simulink model "uavopen_djian"  (R2022b)
settings: Solver=VariableStepAuto  StartTime=0.0  StopTime=50  RelTol=1e-3
libraries: simulink x1
settings Model: Creator=Zzera  LastModifiedBy=Zzera

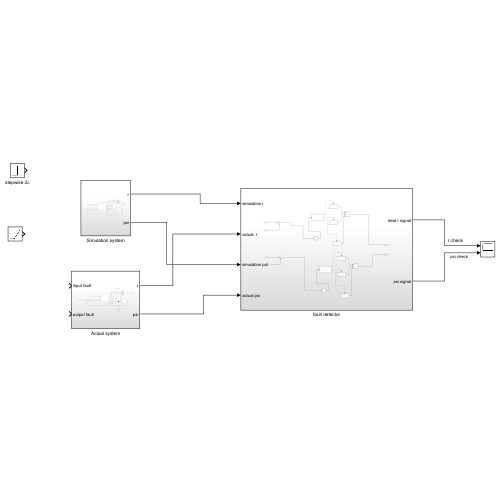
[thumbnail: Simulink's stored preview of the top-level diagram]
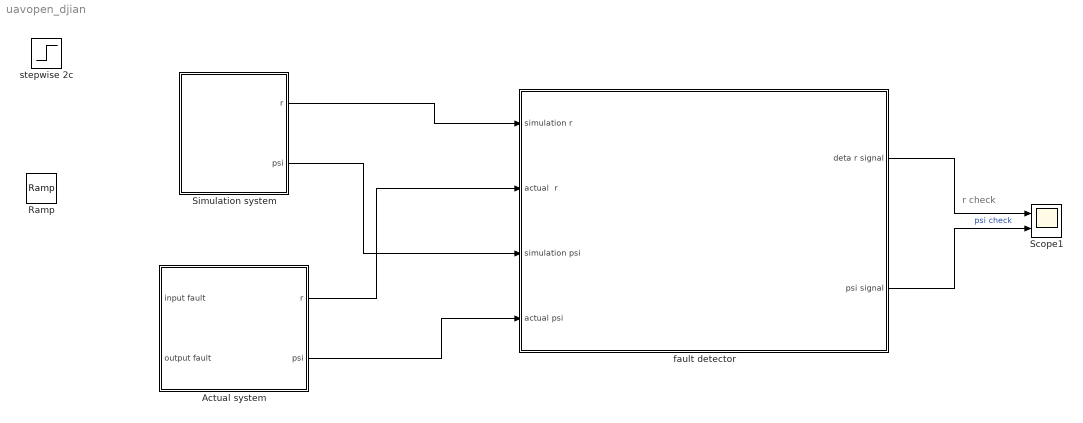
== system uavopen_djian ==
  note: r check
  Actual system : Subsystem
  Ramp : simulink/Sources/Ramp  slope=0.1  start=10  InitialOutput=0
  Scope1 : Scope  NumInputPorts=2
  Simulation system : Subsystem
  fault detector : Subsystem
  stepwise 2c : Step  After=0.2  SampleTime=10
  wires:
  Simulation system/1(" r") -> fault detector/1(simulation r)
  Actual system/1(" r") -> fault detector/2(actual  r)
  Simulation system/2(psi) -> fault detector/3(simulation psi)
  Actual system/2(psi) -> fault detector/4(actual psi)
  fault detector/1(deta r signal) -> Scope1/1
  fault detector/2(psi signal) -> Scope1/2  "psi check"

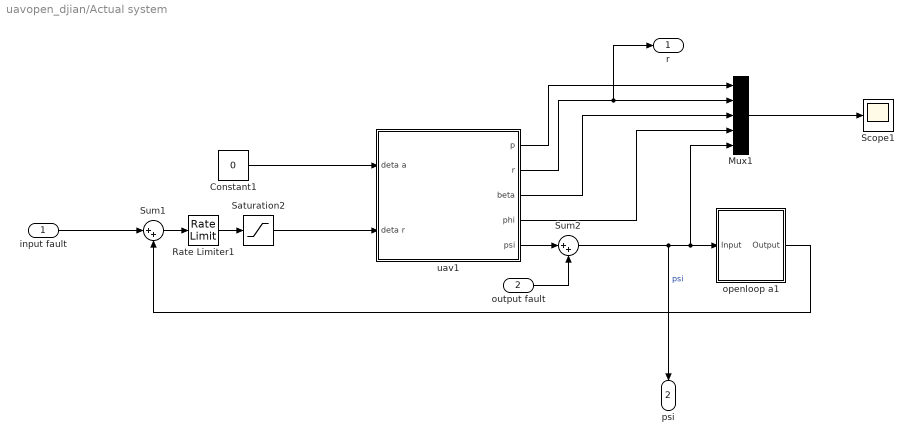
== system uavopen_djian/Actual system ==
  input fault : Inport
  output fault : Inport  Port=2
  Constant1 : Constant  Value=0
  Mux1 : Mux  Inputs=5
  Rate Limiter1 : RateLimiter  RisingSlewLimit=0.3491  FallingSlewLimit=-0.3491
  Saturation2 : Saturate  UpperLimit=1.308  LowerLimit=-1.308
  Scope1 : Scope
  Sum1 : Sum  Inputs=|++
  Sum2 : Sum  Inputs=|++
  openloop a1 : Subsystem
  uav1 : Subsystem
  " r" : Outport
  psi : Outport  Port=2
  wires:
  Sum2/1 -> psi/1, Mux1/5, openloop a1/1(Input)  "psi"
  Saturation2/1 -> uav1/2(deta r)
  openloop a1/1(Output) -> Sum1/2
  uav1/2(r) -> " r"/1, Mux1/2
  uav1/4(phi) -> Mux1/4
  Rate Limiter1/1 -> Saturation2/1
  uav1/1(p) -> Mux1/1
  output fault/1 -> Sum2/2
  Mux1/1 -> Scope1/1
  Constant1/1 -> uav1/1(deta a)
  uav1/3(beta) -> Mux1/3
  Sum1/1 -> Rate Limiter1/1
  uav1/5(psi) -> Sum2/1
  input fault/1 -> Sum1/1

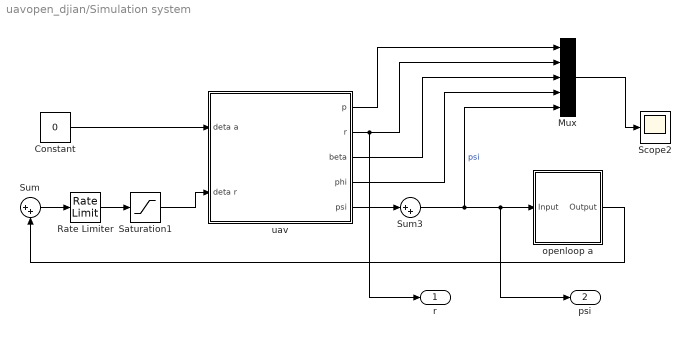
== system uavopen_djian/Simulation system ==
  Constant : Constant  Value=0
  Mux : Mux  Inputs=5
  Rate Limiter : RateLimiter  RisingSlewLimit=0.3491  FallingSlewLimit=-0.3491
  Saturation1 : Saturate  UpperLimit=1.308  LowerLimit=-1.308
  Scope2 : Scope
  Sum : Sum  Inputs=|++
  Sum3 : Sum  Inputs=|++
  openloop a : Subsystem
  uav : Subsystem
  " r" : Outport
  psi : Outport  Port=2
  wires:
  uav/4(phi) -> Mux/4
  uav/5(psi) -> Sum3/1
  Sum3/1 -> psi/1, openloop a/1(Input), Mux/5  "psi"
  Saturation1/1 -> uav/2(deta r)
  uav/2(r) -> " r"/1, Mux/2
  uav/1(p) -> Mux/1
  Rate Limiter/1 -> Saturation1/1
  uav/3(beta) -> Mux/3
  openloop a/1(Output) -> Sum/2
  Mux/1 -> Scope2/1
  Constant/1 -> uav/1(deta a)
  Sum/1 -> Rate Limiter/1

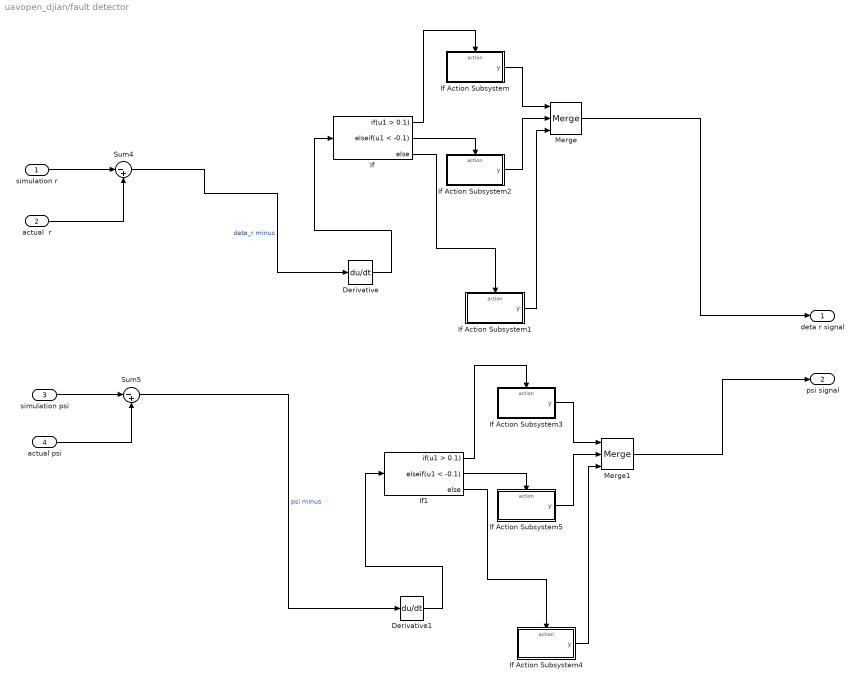
== system uavopen_djian/fault detector ==
  simulation r : Inport
  actual  r : Inport  Port=2
  simulation psi : Inport  Port=3
  actual psi : Inport  Port=4
  Derivative : Derivative
  Derivative1 : Derivative
  If : If  IfExpression=u1 > 0.1  ElseIfExpressions=u1 < -0.1  ZeroCross=off
  If Action Subsystem : Subsystem  TreatAsAtomicUnit=on
  If Action Subsystem1 : Subsystem  TreatAsAtomicUnit=on
  If Action Subsystem2 : Subsystem  TreatAsAtomicUnit=on
  If Action Subsystem3 : Subsystem  TreatAsAtomicUnit=on
  If Action Subsystem4 : Subsystem  TreatAsAtomicUnit=on
  If Action Subsystem5 : Subsystem  TreatAsAtomicUnit=on
  If1 : If  IfExpression=u1 > 0.1  ElseIfExpressions=u1 < -0.1  ZeroCross=off
  Merge : Merge  Inputs=3
  Merge1 : Merge  Inputs=3
  Sum4 : Sum  Inputs=|-+
  Sum5 : Sum  Inputs=|-+
  deta r signal : Outport
  psi signal : Outport  Port=2
  wires:
  If Action Subsystem3/1(y) -> Merge1/1
  If/3 -> If Action Subsystem1/Action
  Derivative/1 -> If/1
  If Action Subsystem/1(y) -> Merge/1
  Derivative1/1 -> If1/1
  If Action Subsystem5/1(y) -> Merge1/2
  If Action Subsystem4/1(y) -> Merge1/3
  simulation r/1 -> Sum4/1
  If1/1 -> If Action Subsystem3/Action
  If1/3 -> If Action Subsystem4/Action
  If1/2 -> If Action Subsystem5/Action
  If/2 -> If Action Subsystem2/Action
  Sum4/1 -> Derivative/1  "deta_r minus"
  Merge1/1 -> psi signal/1
  If/1 -> If Action Subsystem/Action
  If Action Subsystem2/1(y) -> Merge/2
  If Action Subsystem1/1(y) -> Merge/3
  Sum5/1 -> Derivative1/1  "psi minus"
  Merge/1 -> deta r signal/1
  actual  r/1 -> Sum4/2
  simulation psi/1 -> Sum5/1
  actual psi/1 -> Sum5/2

== system uavopen_djian/Actual system/openloop a1 ==
  Input : Inport
  If : If  IfExpression=u1>0.1746  ElseIfExpressions=u1<-0.1745  ShowElse=off
  If Action Subsystem : Subsystem  TreatAsAtomicUnit=on
  If Action Subsystem1 : Subsystem  TreatAsAtomicUnit=on
  Merge : Merge  InitialOutput=[0.3491]
  Output : Outport
  wires:
  Input/1 -> If/1
  If Action Subsystem/1(y) -> Merge/1
  If Action Subsystem1/1(Out1) -> Merge/2
  If/1 -> If Action Subsystem/Action
  If/2 -> If Action Subsystem1/Action
  Merge/1 -> Output/1

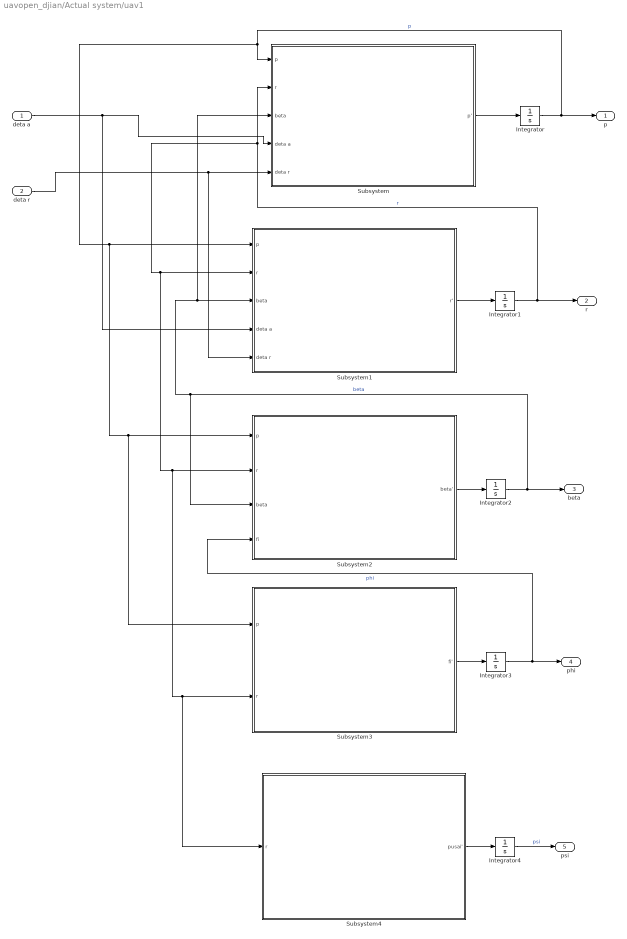
== system uavopen_djian/Actual system/uav1 ==
  deta a : Inport
  deta r : Inport  Port=2
  Integrator{,1..4} (5 alike) : Integrator
  Subsystem : Subsystem
  Subsystem1 : Subsystem
  Subsystem2 : Subsystem
  Subsystem3 : Subsystem
  Subsystem4 : Subsystem
  p : Outport
  r : Outport  Port=2
  beta : Outport  Port=3
  phi : Outport  Port=4
  psi : Outport  Port=5
  wires:
  Integrator4/1 -> psi/1  "psi"
  Integrator3/1 -> phi/1, Subsystem2/4(fi)  "phi"
  Subsystem/1(p') -> Integrator/1
  Subsystem3/1(fi') -> Integrator3/1
  Integrator/1 -> p/1, Subsystem3/1(p), Subsystem2/1(p), Subsystem1/1(p), Subsystem/1(p)  "p"
  Subsystem2/1(beta') -> Integrator2/1
  Integrator1/1 -> r/1, Subsystem/2(r), Subsystem4/1(r), Subsystem3/2(r), Subsystem2/2(r), Subsystem1/2(r)  "r"
  Subsystem4/1(pusai') -> Integrator4/1
  Integrator2/1 -> beta/1, Subsystem2/3(beta), Subsystem/3(beta), Subsystem1/3(beta)  "beta"
  Subsystem1/1(r') -> Integrator1/1
  deta a/1 -> Subsystem1/4(deta a), Subsystem/4(deta a)
  deta r/1 -> Subsystem1/5(deta r), Subsystem/5(deta r)

== system uavopen_djian/Simulation system/openloop a ==
  Input : Inport
  If : If  IfExpression=u1>0.1746  ElseIfExpressions=u1<-0.1745  ShowElse=off
  If Action Subsystem : Subsystem  TreatAsAtomicUnit=on
  If Action Subsystem1 : Subsystem  TreatAsAtomicUnit=on
  Merge : Merge  InitialOutput=[0.3491]
  Output : Outport
  wires:
  Input/1 -> If/1
  If Action Subsystem/1(y) -> Merge/1
  If Action Subsystem1/1(Out1) -> Merge/2
  If/1 -> If Action Subsystem/Action
  If/2 -> If Action Subsystem1/Action
  Merge/1 -> Output/1

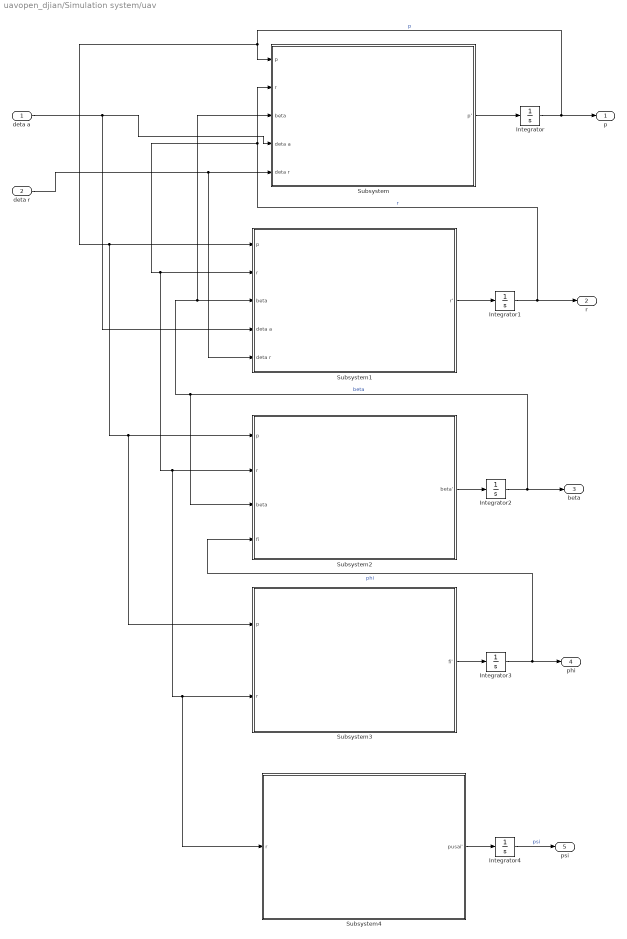
== system uavopen_djian/Simulation system/uav ==
  deta a : Inport
  deta r : Inport  Port=2
  Integrator{,1..4} (5 alike) : Integrator
  Subsystem : Subsystem
  Subsystem1 : Subsystem
  Subsystem2 : Subsystem
  Subsystem3 : Subsystem
  Subsystem4 : Subsystem
  p : Outport
  r : Outport  Port=2
  beta : Outport  Port=3
  phi : Outport  Port=4
  psi : Outport  Port=5
  wires:
  Integrator4/1 -> psi/1  "psi"
  Integrator3/1 -> phi/1, Subsystem2/4(fi)  "phi"
  Subsystem/1(p') -> Integrator/1
  Subsystem3/1(fi') -> Integrator3/1
  Integrator/1 -> p/1, Subsystem3/1(p), Subsystem2/1(p), Subsystem1/1(p), Subsystem/1(p)  "p"
  Subsystem2/1(beta') -> Integrator2/1
  Integrator1/1 -> r/1, Subsystem/2(r), Subsystem4/1(r), Subsystem3/2(r), Subsystem2/2(r), Subsystem1/2(r)  "r"
  Subsystem4/1(pusai') -> Integrator4/1
  Integrator2/1 -> beta/1, Subsystem2/3(beta), Subsystem/3(beta), Subsystem1/3(beta)  "beta"
  Subsystem1/1(r') -> Integrator1/1
  deta a/1 -> Subsystem1/4(deta a), Subsystem/4(deta a)
  deta r/1 -> Subsystem1/5(deta r), Subsystem/5(deta r)

== system uavopen_djian/fault detector/If Action Subsystem ==
  Action Port : ActionPort  ActionPortLabel=if(u1 > 0.1)
  Constant : Constant
  y : Outport
  wires:
  Constant/1 -> y/1

== system uavopen_djian/fault detector/If Action Subsystem1 ==
  Action Port : ActionPort  ActionPortLabel=else
  Constant : Constant  Value=0
  y : Outport
  wires:
  Constant/1 -> y/1

== system uavopen_djian/fault detector/If Action Subsystem2 ==
  Action Port : ActionPort  ActionPortLabel=elseif(u1 < -0.1)
  Constant : Constant
  y : Outport
  wires:
  Constant/1 -> y/1

== system uavopen_djian/fault detector/If Action Subsystem3 ==
  Action Port : ActionPort  ActionPortLabel=if(u1 > 0.1)
  Constant : Constant
  y : Outport
  wires:
  Constant/1 -> y/1

== system uavopen_djian/fault detector/If Action Subsystem4 ==
  Action Port : ActionPort  ActionPortLabel=else
  Constant : Constant  Value=0
  y : Outport
  wires:
  Constant/1 -> y/1

== system uavopen_djian/fault detector/If Action Subsystem5 ==
  Action Port : ActionPort  ActionPortLabel=elseif(u1 < -0.1)
  Constant : Constant
  y : Outport
  wires:
  Constant/1 -> y/1

== system uavopen_djian/Actual system/openloop a1/If Action Subsystem ==
  Action Port : ActionPort  ActionPortLabel=if(u1>0.1746)
  Constant : Constant  Value=-0.3491
  y : Outport
  wires:
  Constant/1 -> y/1

== system uavopen_djian/Actual system/openloop a1/If Action Subsystem1 ==
  Action Port : ActionPort  ActionPortLabel=elseif(u1<-0.1745)
  Constant : Constant  Value=0.3491
  Out1 : Outport
  wires:
  Constant/1 -> Out1/1

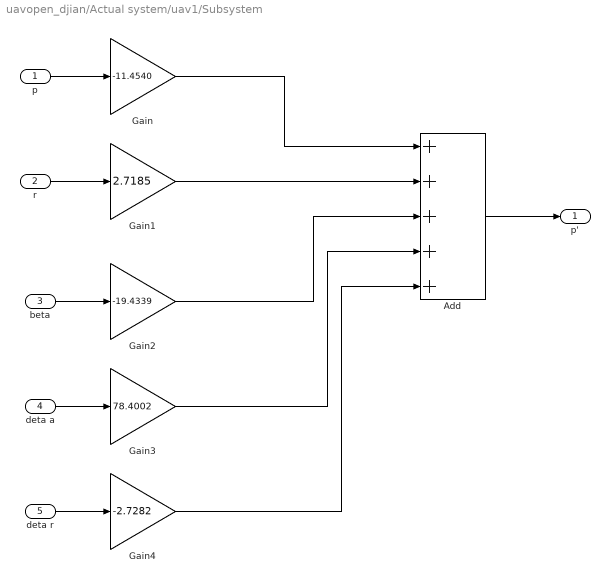
== system uavopen_djian/Actual system/uav1/Subsystem ==
  p : Inport
  r : Inport  Port=2
  beta : Inport  Port=3
  deta a : Inport  Port=4
  deta r : Inport  Port=5
  Add : Sum  Inputs=+++++
  Gain : Gain  Gain=-11.4540
  Gain1 : Gain  Gain=2.7185
  Gain2 : Gain  Gain=-19.4339
  Gain3 : Gain  Gain=78.4002
  Gain4 : Gain  Gain=-2.7282
  p' : Outport
  wires:
  Gain2/1 -> Add/3
  Gain3/1 -> Add/4
  Gain/1 -> Add/1
  Gain1/1 -> Add/2
  Gain4/1 -> Add/5
  p/1 -> Gain/1
  r/1 -> Gain1/1
  beta/1 -> Gain2/1
  deta a/1 -> Gain3/1
  deta r/1 -> Gain4/1
  Add/1 -> p'/1

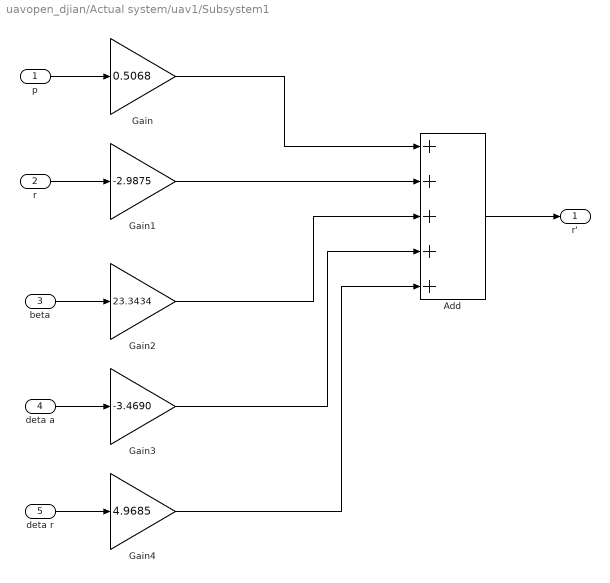
== system uavopen_djian/Actual system/uav1/Subsystem1 ==
  p : Inport
  r : Inport  Port=2
  beta : Inport  Port=3
  deta a : Inport  Port=4
  deta r : Inport  Port=5
  Add : Sum  Inputs=+++++
  Gain : Gain  Gain=0.5068
  Gain1 : Gain  Gain=-2.9875
  Gain2 : Gain  Gain=23.3434
  Gain3 : Gain  Gain=-3.4690
  Gain4 : Gain  Gain=4.9685
  r' : Outport
  wires:
  p/1 -> Gain/1
  Gain4/1 -> Add/5
  Gain1/1 -> Add/2
  Gain/1 -> Add/1
  Gain2/1 -> Add/3
  beta/1 -> Gain2/1
  Gain3/1 -> Add/4
  deta a/1 -> Gain3/1
  Add/1 -> r'/1
  deta r/1 -> Gain4/1
  r/1 -> Gain1/1

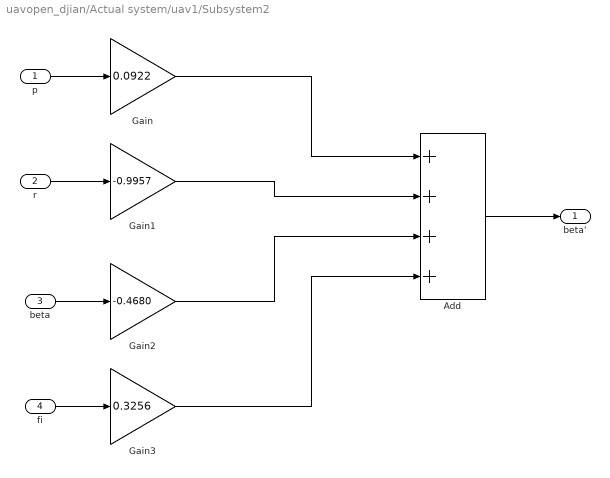
== system uavopen_djian/Actual system/uav1/Subsystem2 ==
  p : Inport
  r : Inport  Port=2
  beta : Inport  Port=3
  fi : Inport  Port=4
  Add : Sum  Inputs=++++
  Gain : Gain  Gain=0.0922
  Gain1 : Gain  Gain=-0.9957
  Gain2 : Gain  Gain=-0.4680
  Gain3 : Gain  Gain=0.3256
  beta' : Outport
  wires:
  p/1 -> Gain/1
  Gain1/1 -> Add/2
  Gain/1 -> Add/1
  Gain2/1 -> Add/3
  beta/1 -> Gain2/1
  Gain3/1 -> Add/4
  fi/1 -> Gain3/1
  Add/1 -> beta'/1
  r/1 -> Gain1/1

== system uavopen_djian/Actual system/uav1/Subsystem3 ==
  p : Inport
  r : Inport  Port=2
  Add : Sum
  Gain : Gain
  Gain1 : Gain  Gain=0.0926
  fi' : Outport
  wires:
  p/1 -> Gain/1
  Gain1/1 -> Add/2
  Gain/1 -> Add/1
  Add/1 -> fi'/1
  r/1 -> Gain1/1

== system uavopen_djian/Actual system/uav1/Subsystem4 ==
  r : Inport
  Gain1 : Gain
  pusai' : Outport
  wires:
  r/1 -> Gain1/1
  Gain1/1 -> pusai'/1

== system uavopen_djian/Simulation system/openloop a/If Action Subsystem ==
  Action Port : ActionPort  ActionPortLabel=if(u1>0.1746)
  Constant : Constant  Value=-0.3491
  y : Outport
  wires:
  Constant/1 -> y/1

== system uavopen_djian/Simulation system/openloop a/If Action Subsystem1 ==
  Action Port : ActionPort  ActionPortLabel=elseif(u1<-0.1745)
  Constant : Constant  Value=0.3491
  Out1 : Outport
  wires:
  Constant/1 -> Out1/1

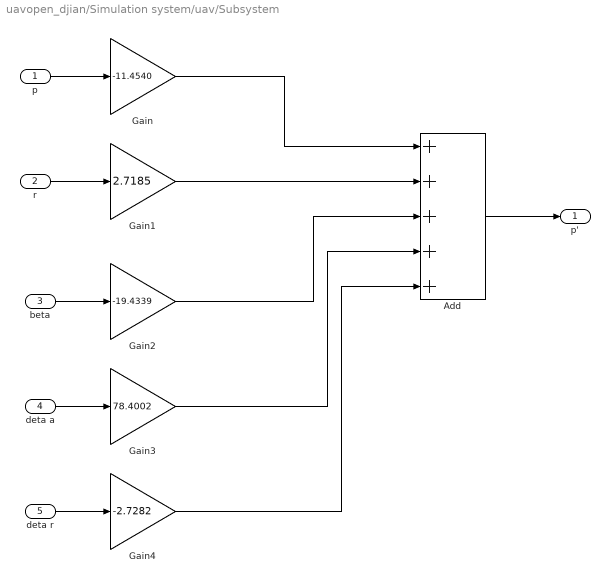
== system uavopen_djian/Simulation system/uav/Subsystem ==
  p : Inport
  r : Inport  Port=2
  beta : Inport  Port=3
  deta a : Inport  Port=4
  deta r : Inport  Port=5
  Add : Sum  Inputs=+++++
  Gain : Gain  Gain=-11.4540
  Gain1 : Gain  Gain=2.7185
  Gain2 : Gain  Gain=-19.4339
  Gain3 : Gain  Gain=78.4002
  Gain4 : Gain  Gain=-2.7282
  p' : Outport
  wires:
  Gain2/1 -> Add/3
  Gain3/1 -> Add/4
  Gain/1 -> Add/1
  Gain1/1 -> Add/2
  Gain4/1 -> Add/5
  p/1 -> Gain/1
  r/1 -> Gain1/1
  beta/1 -> Gain2/1
  deta a/1 -> Gain3/1
  deta r/1 -> Gain4/1
  Add/1 -> p'/1

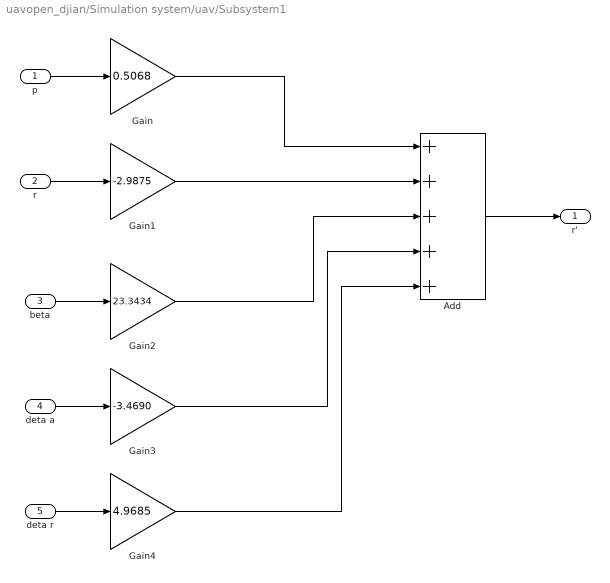
== system uavopen_djian/Simulation system/uav/Subsystem1 ==
  p : Inport
  r : Inport  Port=2
  beta : Inport  Port=3
  deta a : Inport  Port=4
  deta r : Inport  Port=5
  Add : Sum  Inputs=+++++
  Gain : Gain  Gain=0.5068
  Gain1 : Gain  Gain=-2.9875
  Gain2 : Gain  Gain=23.3434
  Gain3 : Gain  Gain=-3.4690
  Gain4 : Gain  Gain=4.9685
  r' : Outport
  wires:
  p/1 -> Gain/1
  Gain4/1 -> Add/5
  Gain1/1 -> Add/2
  Gain/1 -> Add/1
  Gain2/1 -> Add/3
  beta/1 -> Gain2/1
  Gain3/1 -> Add/4
  deta a/1 -> Gain3/1
  Add/1 -> r'/1
  deta r/1 -> Gain4/1
  r/1 -> Gain1/1

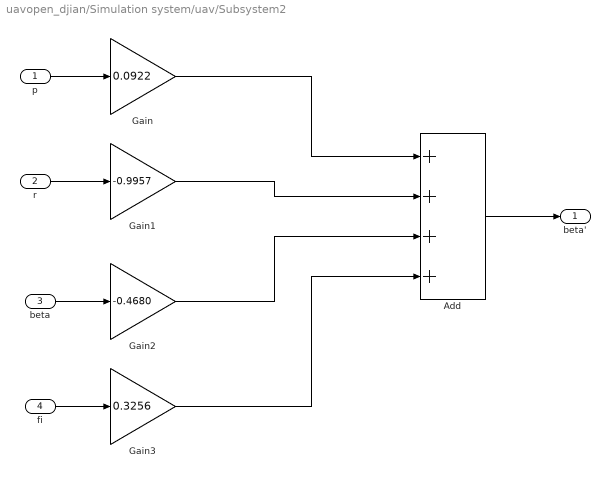
== system uavopen_djian/Simulation system/uav/Subsystem2 ==
  p : Inport
  r : Inport  Port=2
  beta : Inport  Port=3
  fi : Inport  Port=4
  Add : Sum  Inputs=++++
  Gain : Gain  Gain=0.0922
  Gain1 : Gain  Gain=-0.9957
  Gain2 : Gain  Gain=-0.4680
  Gain3 : Gain  Gain=0.3256
  beta' : Outport
  wires:
  p/1 -> Gain/1
  Gain1/1 -> Add/2
  Gain/1 -> Add/1
  Gain2/1 -> Add/3
  beta/1 -> Gain2/1
  Gain3/1 -> Add/4
  fi/1 -> Gain3/1
  Add/1 -> beta'/1
  r/1 -> Gain1/1

== system uavopen_djian/Simulation system/uav/Subsystem3 ==
  p : Inport
  r : Inport  Port=2
  Add : Sum
  Gain : Gain
  Gain1 : Gain  Gain=0.0926
  fi' : Outport
  wires:
  p/1 -> Gain/1
  Gain1/1 -> Add/2
  Gain/1 -> Add/1
  Add/1 -> fi'/1
  r/1 -> Gain1/1

== system uavopen_djian/Simulation system/uav/Subsystem4 ==
  r : Inport
  Gain1 : Gain
  pusai' : Outport
  wires:
  r/1 -> Gain1/1
  Gain1/1 -> pusai'/1
